simulink model "test_LTI"  (R2021b)
settings: Solver=FixedStepDiscrete  StartTime=0.0  StopTime=10  FixedStep=Ts  MaxStep=Tc  RelTol=1e-3
values from neighbouring files (symbols this model uses):
  tau = 2    [script.m]
undefined symbols (not defined in the file or in its folder): R1, R2
settings Model: Creator=francesco  LastModifiedBy=antony
settings SolverCC: AlgebraicLoopSolver=TrustRegion
settings DataIOCC: ReturnWorkspaceOutputs=off
settings OptimizationCC: LifeSpan=inf
settings DebuggingCC: SFExecutionAtInitializationDiag=none  SFMachineParentedDataDiag=warning  ArithmeticOperatorsInVariantConditions=warning
settings HardwareCC: ProdBitPerSizeT=32  ProdBitPerPtrDiffT=32  ProdWordSize=32  ProdHWDeviceType=Specified
settings SFSimCC: SimUseLocalCustomCode=off  CustomCodeUndefinedFunction=UseInterfaceOnly
settings RTWCC: RTWUseLocalCustomCode=off
settings CodeAppCC: StateflowObjectComments=on

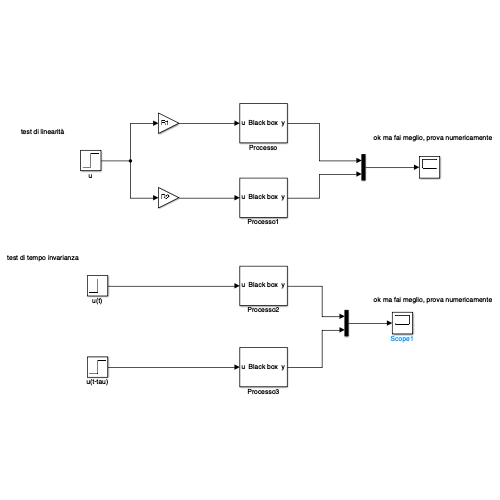
[thumbnail: Simulink's stored preview of the top-level diagram]
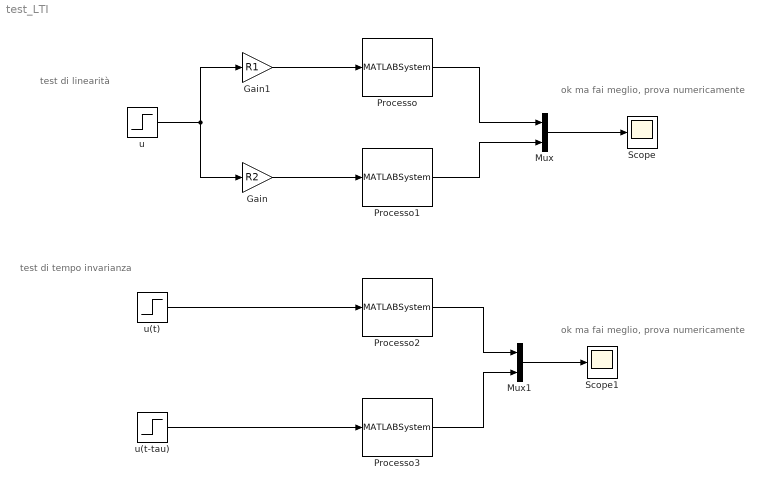
== system test_LTI ==
  note: test di tempo invarianza
  note: test di linearità
  note: ok ma fai meglio, prova numericamente
  note: ok ma fai meglio, prova numericamente
  Gain : Gain  Gain=R2
  Gain1 : Gain  Gain=R1
  Mux : Mux  Inputs=2
  Mux1 : Mux  Inputs=2
  Processo{,1..3} (4 alike) : MATLABSystem  System=linSysObj  SimulateUsing=Interpreted execution
      mask Type: linSysObj
      mask Display:
      | disp('Black box');
      | port_label('input',1,'u');
      | port_label('output',1,'y');
  Scope : Scope
  Scope1 : Scope
  u : Step  Time=0  SampleTime=0.01
  u(t) : Step  Time=0  SampleTime=0.01
  u(t-tau) : Step  Time=tau  SampleTime=0.01
  wires:
  u/1 -> Gain1/1, Gain/1
  Gain1/1 -> Processo/1
  Gain/1 -> Processo1/1
  Processo/1 -> Mux/1
  Processo1/1 -> Mux/2
  Mux/1 -> Scope/1
  Mux1/1 -> Scope1/1
  Processo3/1 -> Mux1/2
  Processo2/1 -> Mux1/1
  u(t)/1 -> Processo2/1
  u(t-tau)/1 -> Processo3/1
